simulink model "ControlVehicle"  (R2026a)
settings: Solver=FixedStepAuto  StopTime=inf
undefined symbols (not defined in the file or in its folder): fractalcoef, Sim3dSensor
libraries: sensorgpslib x1, mspsensorlib x1, sim3dcameralib x1, sim3dprobsensorlib x1, sim3dautolib x1, sim3dlib x1
(part 2 of 2)

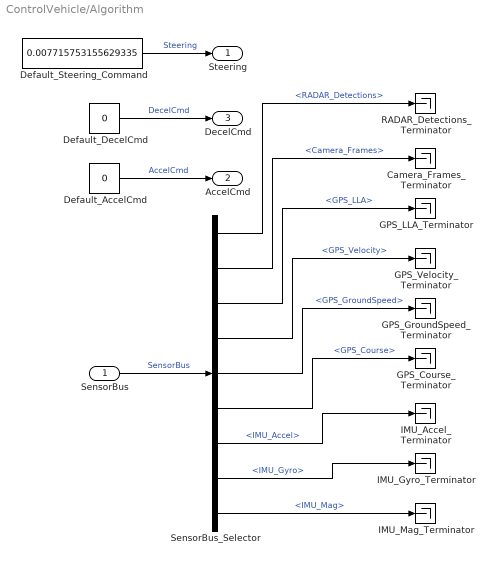
== system ControlVehicle/Algorithm ==
  SensorBus : Inport
  Camera_Frames_Terminator : Terminator
  Default_AccelCmd : Constant  Value=0
  Default_DecelCmd : Constant  Value=0
  Default_Steering_Command : Constant  Value=0.007715753155629335
  GPS_Course_Terminator : Terminator
  GPS_GroundSpeed_Terminator : Terminator
  GPS_LLA_Terminator : Terminator
  GPS_Velocity_Terminator : Terminator
  IMU_Accel_Terminator : Terminator
  IMU_Gyro_Terminator : Terminator
  IMU_Mag_Terminator : Terminator
  RADAR_Detections_Terminator : Terminator
  SensorBus_Selector : BusSelector  OutputSignals=RADAR_Detections,Camera_Frames,GPS_LLA,GPS_Velocity,GPS_GroundSpeed,GPS_Course,IMU_Accel,IMU_Gyro,IMU_Mag
  Steering : Outport
  AccelCmd : Outport  Port=2
  DecelCmd : Outport  Port=3
  wires:
  Default_Steering_Command/1 -> Steering/1  "Steering"
  Default_DecelCmd/1 -> DecelCmd/1  "DecelCmd"
  SensorBus_Selector/2 -> Camera_Frames_Terminator/1  "<Camera_Frames>"
  Default_AccelCmd/1 -> AccelCmd/1  "AccelCmd"
  SensorBus/1 -> SensorBus_Selector/1  "SensorBus"
  SensorBus_Selector/1 -> RADAR_Detections_Terminator/1  "<RADAR_Detections>"
  SensorBus_Selector/3 -> GPS_LLA_Terminator/1  "<GPS_LLA>"
  SensorBus_Selector/4 -> GPS_Velocity_Terminator/1  "<GPS_Velocity>"
  SensorBus_Selector/5 -> GPS_GroundSpeed_Terminator/1  "<GPS_GroundSpeed>"
  SensorBus_Selector/6 -> GPS_Course_Terminator/1  "<GPS_Course>"
  SensorBus_Selector/7 -> IMU_Accel_Terminator/1  "<IMU_Accel>"
  SensorBus_Selector/8 -> IMU_Gyro_Terminator/1  "<IMU_Gyro>"
  SensorBus_Selector/9 -> IMU_Mag_Terminator/1  "<IMU_Mag>"

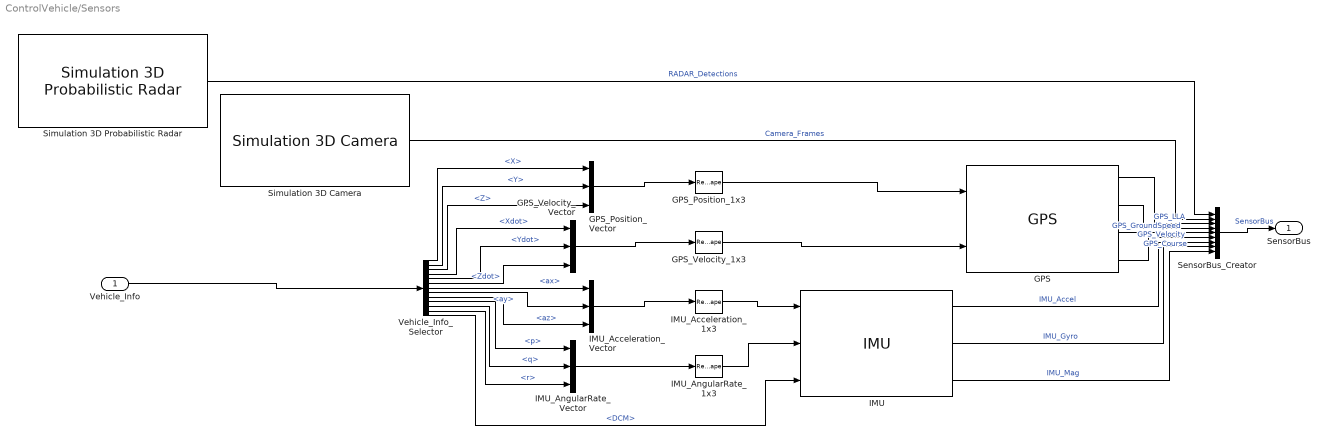
== system ControlVehicle/Sensors ==
  Vehicle_Info : Inport
  GPS : sensorgpslib/GPS  DispRefFrame=NED  PositionInputFormat=Local  ReferenceLocation=[ 0, 0, 0 ]  HorizontalPositionAccuracy=1.6  VerticalPositionAccuracy=3  VelocityAccuracy=0.1  DecayFactor=0.999  SeedDouble=67  SimulateUsing=Interpreted execution
  GPS_Position_1x3 : Reshape  OutputDimensionality=Customize  OutputDimensions=[1 3]
  GPS_Position_Vector : Mux  Inputs=3
  GPS_Velocity_1x3 : Reshape  OutputDimensionality=Customize  OutputDimensions=[1 3]
  GPS_Velocity_Vector : Mux  Inputs=3
  IMU : mspsensorlib/IMU  DispRefFrame=NED  TemperaturePort=off  Temperature=25  MagneticFieldPort=off  MagneticFieldNED=[ 27.5550, -2.4169, -16.0849 ]  MagneticFieldENU=[ -2.4169, 27.5550, 16.0849 ]  SeedDouble=67  SimulateUsing=Interpreted execution  AccelParamsMeasurementRange=Inf  AccelParamsResolution=0  AccelParamsConstantBias=[ 0, 0, 0 ]  AccelParamsAxesMisalignment=[ 100, 0, 0; 0, 100, 0; 0, 0, 100 ]  AccelParamsNoiseDensity=[ 0, 0, 0 ]  AccelParamsBiasInstability=[ 0, 0, 0 ]  AccelParamsBiasInstabilityNumerator=fractalcoef().Numerator  AccelParamsBiasInstabilityDenominator=fractalcoef().Denominator  AccelParamsRandomWalk=[ 0, 0, 0 ]  AccelParamsNoiseType=double-sided  AccelParamsTemperatureBias=[ 0, 0, 0 ]  AccelParamsTemperatureScaleFactor=[ 0, 0, 0 ]  GyroParamsMeasurementRange=Inf  GyroParamsResolution=0  GyroParamsConstantBias=[ 0, 0, 0 ]  GyroParamsAxesMisalignment=[ 100, 0, 0; 0, 100, 0; 0, 0, 100 ]  GyroParamsAccelerationBias=[ 0, 0, 0 ]  GyroParamsNoiseDensity=[ 0, 0, 0 ]  GyroParamsBiasInstability=[ 0, 0, 0 ]  GyroParamsBiasInstabilityNumerator=fractalcoef().Numerator  GyroParamsBiasInstabilityDenominator=fractalcoef().Denominator  GyroParamsRandomWalk=[ 0, 0, 0 ]  GyroParamsNoiseType=double-sided  GyroParamsTemperatureBias=[ 0, 0, 0 ]  GyroParamsTemperatureScaleFactor=[ 0, 0, 0 ]  MagParamsMeasurementRange=Inf  MagParamsResolution=0  MagParamsConstantBias=[ 0, 0, 0 ]  MagParamsAxesMisalignment=[ 100, 0, 0; 0, 100, 0; 0, 0, 100 ]  MagParamsNoiseDensity=[ 0, 0, 0 ]  MagParamsBiasInstability=[ 0, 0, 0 ]  MagParamsBiasInstabilityNumerator=fractalcoef().Numerator  MagParamsBiasInstabilityDenominator=fractalcoef().Denominator  MagParamsRandomWalk=[ 0, 0, 0 ]  MagParamsNoiseType=double-sided  MagParamsTemperatureBias=[ 0, 0, 0 ]  MagParamsTemperatureScaleFactor=[ 0, 0, 0 ]
  IMU_Acceleration_1x3 : Reshape  OutputDimensionality=Customize  OutputDimensions=[1 3]
  IMU_Acceleration_Vector : Mux  Inputs=3
  IMU_AngularRate_1x3 : Reshape  OutputDimensionality=Customize  OutputDimensions=[1 3]
  IMU_AngularRate_Vector : Mux  Inputs=3
  SensorBus_Creator : BusCreator  Inputs=9
  Simulation 3D Camera : sim3dcameralib/Simulation 3D Camera  Priority=1  sensorTag=Sim3dSensor�  sensorId=3  sensorName=Sim3dSensor3  vehTagList={'Custom ...';'MYVehicle';'Scene Origin'}  vehTag=MYVehicle  CoordinateSystem=ISO8855  mountLoc=Rearview mirror  offsetFlag=off  tmountOffset=[0, 0, 0]  extTmount=off  rmountOffset=[0, 0, 0]  extRmount=off  FocalLength=[1109, 1109]  OpticalCenter=[640, 360]  ImageSize=[720, 1280]  RadialDistortion=[0, 0]  TangentialDistortion=[0, 0]  SensorSkew=0  VisualizeFieldOfView=off  FieldOfViewRange=61  DepthOutportEnabled=off  SemanticOutportEnabled=off  TransformOutportEnabled=off  SampleTime=-1  mountPoint=[0.327 0 1.19]  mountOrientation=[0 0 0]  aMode=3  ID=3
      settings: LibrarySourceBlock=drivingsim3d/Simulation 3D Camera
  Simulation 3D Probabilistic Radar : sim3dprobsensorlib/Simulation 3D Probabilistic Radar  Priority=1  sensorTag=Sim3dSensor�  sensorId=4  sensorName=Sim3dSensor4  vehTagList={'Custom ...';'MYVehicle';'Scene Origin'}  vehTag=MYVehicle  mountLoc=Front bumper  offsetFlag=off  tmountOffset=[0, 0, 0]  rmountOffset=[0, 0, 0]  AzimuthResolution=4  ElevationResolution=5  RangeResolution=2.5  RangeRateResolution=0.5  AzimuthBiasFraction=0.1  ElevationBiasFraction=0.1  RangeBiasFraction=0.05  RangeRateBiasFraction=0.05  FieldOfView=[ 20, 5 ]  DetectionRange=[ 1, 150 ]  RangeRateLimits=[ -100, 100 ]  DetectionProbability=0.9  FalseAlarmRate=1e-6  ReferenceRange=100  ReferenceRCS=0  HasElevation=on  HasRangeRate=on  HasNoise=on  HasFalseAlarms=on  InitialSeedSource=Repeatable  InitialSeed=0  MaxNumDetections=50  DetectionCoordinates=Ego Cartesian  SpecifyOutputBusName=off  BusName=BusSimulation3DRadarTruthSensor  SampleTime=-1  mountPoint=[2.4735 0 0.44]  mountOrientation=[0 0 0]  aMode=3  ID=4
      settings: LibrarySourceBlock=drivingsim3d/Simulation 3D Probabilistic Radar
  Vehicle_Info_Selector : BusSelector  OutputSignals=InertFrm.Cg.Disp.X,InertFrm.Cg.Disp.Y,InertFrm.Cg.Disp.Z,InertFrm.Cg.Vel.Xdot,InertFrm.Cg.Vel.Ydot,InertFrm.Cg.Vel.Zdot,BdyFrm.Cg.Acc.ax,BdyFrm.Cg.Acc.ay,BdyFrm.Cg.Acc.az,BdyFrm.Cg.AngVel.p,BdyFrm.Cg.AngVel.q,BdyFrm.Cg.AngVel.r,BdyFrm.Cg.DCM
  SensorBus : Outport
  wires:
  SensorBus_Creator/1 -> SensorBus/1  "SensorBus"
  IMU/3 -> SensorBus_Creator/9  "IMU_Mag"
  IMU/2 -> SensorBus_Creator/8  "IMU_Gyro"
  IMU/1 -> SensorBus_Creator/7  "IMU_Accel"
  GPS/4 -> SensorBus_Creator/6  "GPS_Course"
  GPS/3 -> SensorBus_Creator/5  "GPS_GroundSpeed"
  GPS/2 -> SensorBus_Creator/4  "GPS_Velocity"
  GPS/1 -> SensorBus_Creator/3  "GPS_LLA"
  Simulation 3D Camera/1 -> SensorBus_Creator/2  "Camera_Frames"
  Simulation 3D Probabilistic Radar/1 -> SensorBus_Creator/1  "RADAR_Detections"
  IMU_AngularRate_Vector/1 -> IMU_AngularRate_1x3/1
  IMU_Acceleration_Vector/1 -> IMU_Acceleration_1x3/1
  Vehicle_Info_Selector/12 -> IMU_AngularRate_Vector/3  "<r>"
  Vehicle_Info_Selector/11 -> IMU_AngularRate_Vector/2  "<q>"
  Vehicle_Info_Selector/10 -> IMU_AngularRate_Vector/1  "<p>"
  Vehicle_Info_Selector/9 -> IMU_Acceleration_Vector/3  "<az>"
  Vehicle_Info_Selector/8 -> IMU_Acceleration_Vector/2  "<ay>"
  Vehicle_Info_Selector/7 -> IMU_Acceleration_Vector/1  "<ax>"
  GPS_Velocity_Vector/1 -> GPS_Velocity_1x3/1
  GPS_Position_Vector/1 -> GPS_Position_1x3/1
  Vehicle_Info_Selector/6 -> GPS_Velocity_Vector/3  "<Zdot>"
  Vehicle_Info_Selector/5 -> GPS_Velocity_Vector/2  "<Ydot>"
  Vehicle_Info_Selector/4 -> GPS_Velocity_Vector/1  "<Xdot>"
  Vehicle_Info_Selector/3 -> GPS_Position_Vector/3  "<Z>"
  Vehicle_Info_Selector/2 -> GPS_Position_Vector/2  "<Y>"
  Vehicle_Info_Selector/1 -> GPS_Position_Vector/1  "<X>"
  Vehicle_Info/1 -> Vehicle_Info_Selector/1
  GPS_Position_1x3/1 -> GPS/1
  GPS_Velocity_1x3/1 -> GPS/2
  IMU_Acceleration_1x3/1 -> IMU/1
  IMU_AngularRate_1x3/1 -> IMU/2
  Vehicle_Info_Selector/13 -> IMU/3  "<DCM>"
